simulink model "star"  (R2019a)
settings: Solver=FixedStepAuto  StartTime=0.0  StopTime=40  FixedStep=1e-4  RelTol=1e-3
libraries: simulink x2, simulink_extras x1
settings Model: Creator=ogure  LastModifiedBy=ogure
settings DebuggingCC: ArithmeticOperatorsInVariantConditions=warning

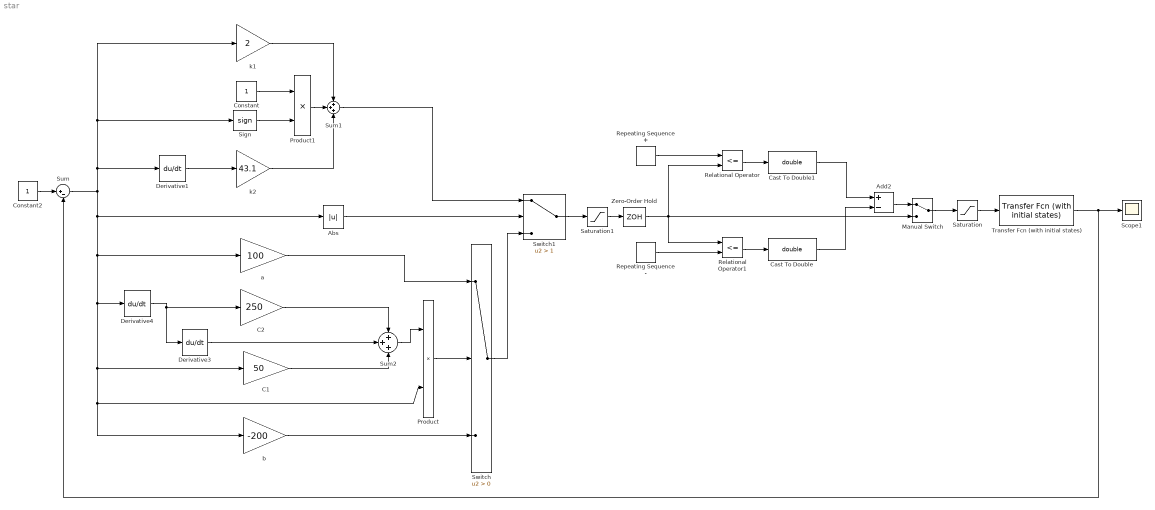
== system star ==
  Abs : Abs
  Add2 : Sum  Inputs=+-
  C1 : Gain  Gain=50
  C2 : Gain  Gain=250
  Cast To Double : DataTypeConversion  OutDataTypeStr=double
  Cast To Double1 : DataTypeConversion  OutDataTypeStr=double
  Constant : Constant
  Constant2 : Constant
  Derivative1 : Derivative  CoefficientInTFapproximation=0.00000001
  Derivative3 : Derivative  CoefficientInTFapproximation=0.00000001
  Derivative4 : Derivative  CoefficientInTFapproximation=0.00000001
  Manual Switch : ManualSwitch
  Product : Product
  Product1 : Product
  Relational Operator : RelationalOperator  Operator=<=  OutDataTypeStr=boolean  ZeroCross=off  RndMeth=Simplest
  Relational Operator1 : RelationalOperator  Operator=<=  OutDataTypeStr=boolean  ZeroCross=off  RndMeth=Simplest
  Repeating Sequence + : simulink/Sources/Repeating Sequence  rep_seq_t=[0 0.01]  rep_seq_y=[0 0.6]
  Repeating Sequence - : simulink/Sources/Repeating Sequence  rep_seq_t=[0 0.01]  rep_seq_y=[0 -0.6]
  Saturation : Saturate  UpperLimit=0.6  LowerLimit=-0.6
  Saturation1 : Saturate  UpperLimit=0.6  LowerLimit=-0.6
  Scope1 : Scope
  Sign : Signum
  Sum : Sum  Inputs=|+-
  Sum1 : Sum  Inputs=+++
  Sum2 : Sum  Inputs=+++
  Switch : Switch  Criteria=u2 > Threshold  ZeroCross=off
  Switch1 : Switch  Criteria=u2 > Threshold  Threshold=1  ZeroCross=off
  Transfer Fcn (with initial states) : simulink_extras/Additional Linear/Transfer Fcn (with initial states)  N=3  D=[9^2 2*6*9 1 0]  X0=[0 0 0]
  Zero-Order Hold : ZeroOrderHold  SampleTime=0.01
  a : Gain  Gain=100
  b : Gain  Gain=-200
  k1 : Gain  Gain=2
  k2 : Gain  Gain=43.1
  wires:
  Constant2/1 -> Sum/1
  Abs/1 -> Switch1/2
  Switch/1 -> Switch1/3
  Sign/1 -> Product1/2
  Constant/1 -> Product1/1
  Product1/1 -> Sum1/2
  Sum1/1 -> Switch1/1
  k1/1 -> Sum1/1
  a/1 -> Switch/1
  b/1 -> Switch/3
  Product/1 -> Switch/2
  Derivative4/1 -> C2/1, Derivative3/1
  C2/1 -> Sum2/1
  C1/1 -> Sum2/3
  Derivative3/1 -> Sum2/2
  Sum2/1 -> Product/1
  Sum/1 -> Derivative1/1, k1/1, Sign/1, Abs/1, b/1, Product/2, C1/1, Derivative4/1, a/1
  k2/1 -> Sum1/3
  Derivative1/1 -> k2/1
  Manual Switch/1 -> Saturation/1
  Saturation/1 -> Transfer Fcn (with initial states)/1
  Transfer Fcn (with initial states)/1 -> Sum/2, Scope1/1
  Relational Operator1/1 -> Cast To Double/1
  Cast To Double/1 -> Add2/2
  Relational Operator/1 -> Cast To Double1/1
  Switch1/1 -> Saturation1/1
  Add2/1 -> Manual Switch/1
  Saturation1/1 -> Zero-Order Hold/1
  Zero-Order Hold/1 -> Relational Operator1/1, Relational Operator/2, Manual Switch/2
  Repeating Sequence +/1 -> Relational Operator/1
  Cast To Double1/1 -> Add2/1
  Repeating Sequence -/1 -> Relational Operator1/2
